simulink library "slip_angle"  (R2025b)
settings: Solver=VariableStepAuto  StartTime=0.0  StopTime=10.0  RelTol=1e-3
settings Model: Creator=alexelliott  LastModifiedBy=alexelliott

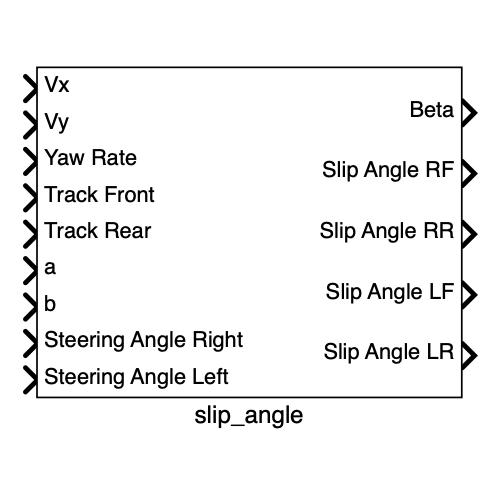
[thumbnail: Simulink's stored preview of the top-level diagram]
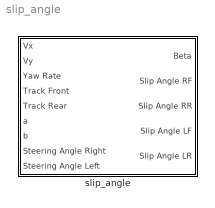
== system slip_angle ==
  slip_angle : Subsystem

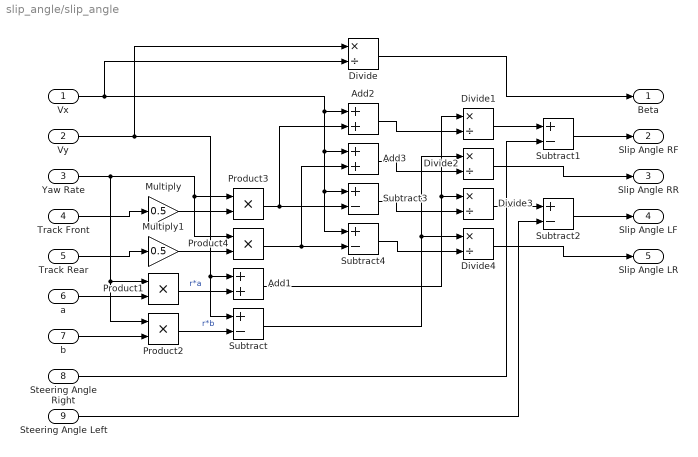
== system slip_angle/slip_angle ==
  Vx : Inport
  Vy : Inport  Port=2
  Yaw Rate : Inport  Port=3
  Track Front : Inport  Port=4
  Track Rear : Inport  Port=5
  a : Inport  Port=6
  b : Inport  Port=7
  Steering Angle Right : Inport  Port=8
  Steering Angle Left : Inport  Port=9
  Add1 : Sum
  Add2 : Sum
  Add3 : Sum
  Divide{,1..4} (5 alike) : Product  Inputs=*/
  Multiply : Gain  Gain=0.5
  Multiply1 : Gain  Gain=0.5
  Product{1..4} (4 alike) : Product
  Subtract{,1..4} (5 alike) : Sum  Inputs=+-
  Beta : Outport
  Slip Angle RF : Outport  Port=2
  Slip Angle RR : Outport  Port=3
  Slip Angle LF : Outport  Port=4
  Slip Angle LR : Outport  Port=5
  wires:
  Steering Angle Left/1 -> Subtract2/2
  Product3/1 -> Subtract3/2, Add2/2
  Product1/1 -> Add1/2  "r*a"
  Multiply/1 -> Product3/2
  Multiply1/1 -> Product4/2
  Subtract1/1 -> Slip Angle RF/1
  Add1/1 -> Divide3/1, Divide1/1
  a/1 -> Product1/2
  Subtract3/1 -> Divide3/2
  Subtract2/1 -> Slip Angle LF/1
  Add3/1 -> Divide2/2
  Track Rear/1 -> Multiply1/1
  Yaw Rate/1 -> Product2/1, Product1/1, Product4/1, Product3/1
  Add2/1 -> Divide1/2
  Vx/1 -> Divide/2, Add2/1, Add3/1, Subtract4/1, Subtract3/1
  Divide1/1 -> Subtract1/1
  Divide2/1 -> Slip Angle RR/1
  Steering Angle Right/1 -> Subtract1/2
  Vy/1 -> Add1/1, Subtract/1, Divide/1
  Divide3/1 -> Subtract2/1
  Product2/1 -> Subtract/2  "r*b"
  Divide/1 -> Beta/1
  Track Front/1 -> Multiply/1
  Subtract/1 -> Divide4/1, Divide2/1
  Subtract4/1 -> Divide4/2
  b/1 -> Product2/2
  Divide4/1 -> Slip Angle LR/1
  Product4/1 -> Subtract4/2, Add3/2
